simulink model "allwheel_standard"  (R2023b)
settings: Solver=VariableStepAuto  StartTime=0.0  StopTime=10.0  RelTol=1e-3
model workspace (MAT data in the model file):
  distfw = 0.0267
  distrw = 0.0267
  wheelrad = 0.004
libraries: mobileRoboticsLib x4
settings Model: Creator=mihai  LastModifiedBy=mihai

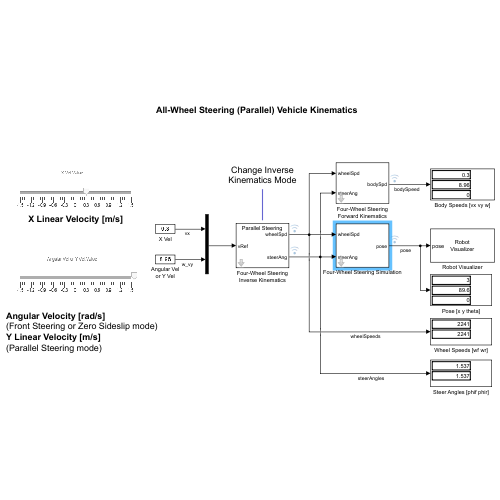
[thumbnail: Simulink's stored preview of the top-level diagram]
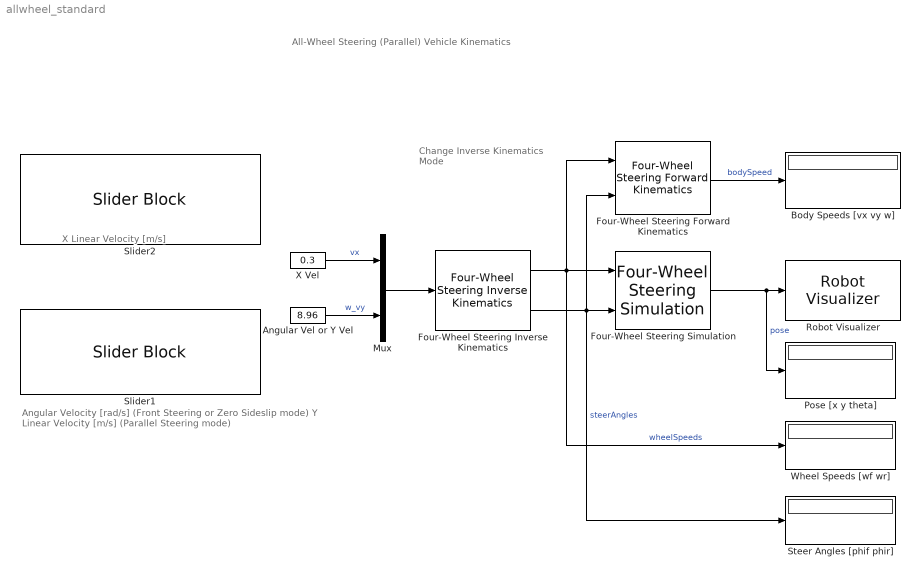
== system allwheel_standard ==
  note: Change Inverse Kinematics Mode
  note: Angular Velocity [rad/s]
      | (Front Steering or Zero Sideslip mode)
      | Y Linear Velocity [m/s]
      | (Parallel Steering mode)
  note: All-Wheel Steering (Parallel) Vehicle Kinematics
  note: X Linear Velocity [m/s]
  Angular Vel or Y Vel : Constant  Value=8.96
  Body Speeds [vx vy w] : Display
  Four-Wheel Steering Forward Kinematics : mobileRoboticsLib/Kinematic Models/Four-Wheel Steering/Four-Wheel Steering Forward Kinematics  wheelRadius=wheelrad  frontWheelDist=distfw  rearWheelDist=distrw
      settings: SourceProductName=Mobile Robotics Simulation Toolbox
  Four-Wheel Steering Inverse Kinematics : mobileRoboticsLib/Kinematic Models/Four-Wheel Steering/Four-Wheel Steering Inverse Kinematics  wheelRadius=wheelrad  frontWheelDist=distfw  rearWheelDist=distrw  ikMode=Parallel Steering
      settings: SourceProductName=Mobile Robotics Simulation Toolbox
  Four-Wheel Steering Simulation : mobileRoboticsLib/Kinematic Models/Four-Wheel Steering/Four-Wheel Steering Simulation  wheelRadius=wheelrad  frontWheelDist=distfw  rearWheelDist=distrw  initX=0  initY=0  initAngle=0  Ts=0.05
      settings: SourceProductName=Mobile Robotics Simulation Toolbox
  Mux : Mux  Inputs=2
  Pose [x y theta] : Display
  Robot Visualizer : mobileRoboticsLib/Environments/Robot Visualizer  Priority=99  robotRadius=0  showTrajectory=on  hasWaypoints=off  hasLidar=off  sensorOffset=[ 0 0 ]  scanAngles=scanAngles  hasObjDetector=off  objDetectorOffset=[ 0, 0 ]  objDetectorAngle=0  objDetectorFOV=pi/4  objDetectorMaxRange=5  objectColors=[ 1, 0, 0; 0, 1, 0; 0, 0, 1 ]  objectMarkers=s
  Slider1 : SliderBlock  ScaleMin=-1.5  ScaleMax=1.5
  Slider2 : SliderBlock  ScaleMin=-1.5  ScaleMax=1.5
  Steer Angles [phif phir] : Display
  Wheel Speeds [wf wr] : Display
  X Vel : Constant  Value=0.3
  wires:
  Four-Wheel Steering Forward Kinematics/1 -> Body Speeds [vx vy w]/1  "bodySpeed"
  Mux/1 -> Four-Wheel Steering Inverse Kinematics/1
  Four-Wheel Steering Inverse Kinematics/2 -> Four-Wheel Steering Forward Kinematics/2, Four-Wheel Steering Simulation/2, Steer Angles [phif phir]/1  "steerAngles"
  Angular Vel or Y Vel/1 -> Mux/2  "w_vy"
  Four-Wheel Steering Inverse Kinematics/1 -> Four-Wheel Steering Forward Kinematics/1, Four-Wheel Steering Simulation/1, Wheel Speeds [wf wr]/1  "wheelSpeeds"
  X Vel/1 -> Mux/1  "vx"
  Four-Wheel Steering Simulation/1 -> Pose [x y theta]/1, Robot Visualizer/1  "pose"
